simulink model "slipm3D_zir"  (R2025b)
settings: Solver=ode4  StartTime=0.0  StopTime=t_stop  FixedStep=t_step  RelTol=1e-3
values from neighbouring files (symbols this model uses):
  dx0 = -0.467    [ref_data_zir.m]
  dy0 = 0.467    [ref_data_zir.m]
  t_step = 0.001    [ref_data_zir.m]
  x0 = 0.151    [ref_data_zir.m]
  y0 = 0.05    [ref_data_zir.m]
settings Model: Creator=Admin  LastModifiedBy=Vishal
settings OptimizationCC: ReuseModelBlockBuffer=off
settings RTWCC: GPUComputeCapability=3.5

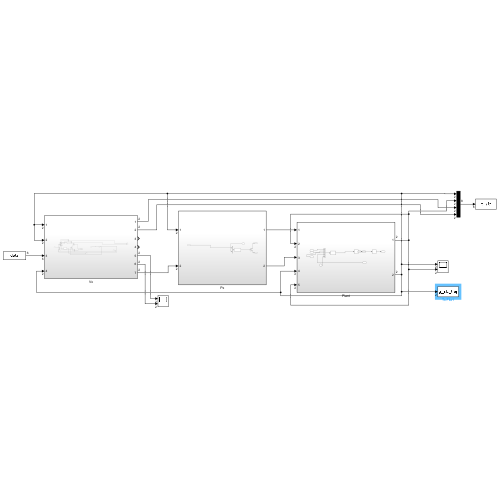
[thumbnail: Simulink's stored preview of the top-level diagram]
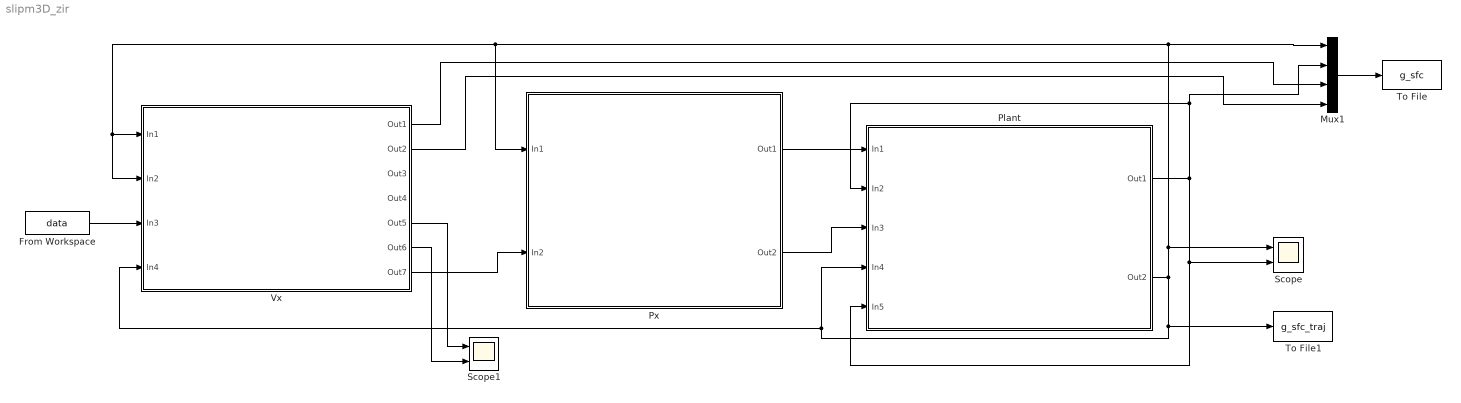
== system slipm3D_zir ==
  From Workspace : FromWorkspace  VariableName=data  OutDataTypeStr=double  SampleTime=t_step
  Mux1 : Mux
  Plant : Subsystem
  Px : Subsystem
  Scope : Scope  NumInputPorts=2
      settings: ActiveDisplayYMinimum=-0.064169644280956978  ActiveDisplayYMaximum=1.077526798528613
  Scope1 : Scope  NumInputPorts=2
      settings: ActiveDisplayYMinimum=0.08202  ActiveDisplayYMaximum=0.48484
  To File : ToFile  Filename=g_sfc  MatrixName=states_sfc
  To File1 : ToFile  Filename=g_sfc_traj  MatrixName=staj
  Vx : Subsystem
  wires:
  Mux1/1 -> To File/1
  Plant/2(Out2) -> To File1/1, Plant/4(In4), Vx/4(In4), Scope/1, Mux1/1, Vx/1(In1), Vx/2(In2), Px/1(In1)
  Plant/1(Out1) -> Plant/5(In5), Scope/2, Plant/2(In2), Mux1/2
  Px/1(Out1) -> Plant/1(In1)
  Px/2(Out2) -> Plant/3(In3)
  From Workspace/1 -> Vx/3(In3)
  Vx/1(Out1) -> Mux1/3
  Vx/2(Out2) -> Mux1/4
  Vx/5(Out5) -> Scope1/1
  Vx/6(Out6) -> Scope1/2
  Vx/7(Out7) -> Px/2(In2)

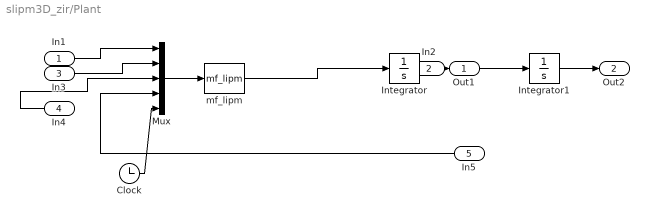
== system slipm3D_zir/Plant ==
  In1 : Inport
  In2 : Inport  Port=2
  In3 : Inport  Port=3
  In4 : Inport  Port=4
  In5 : Inport  Port=5
  Clock : Clock
  Integrator : Integrator  InitialCondition=[dx0,dy0]
  Integrator1 : Integrator  InitialCondition=[x0,y0]
  Mux : Mux  Inputs=5
  mf_lipm : MATLABFcn  MATLABFcn=mf_lipm  OutputDimensions=2
  Out1 : Outport
  Out2 : Outport  Port=2
  wires:
  Clock/1 -> Mux/5
  In4/1 -> Mux/3
  mf_lipm/1 -> Integrator/1
  Integrator/1 -> Out1/1
  In1/1 -> Mux/1
  Integrator1/1 -> Out2/1
  Mux/1 -> mf_lipm/1
  In3/1 -> Mux/2
  In5/1 -> Mux/4
  In2/1 -> Integrator1/1

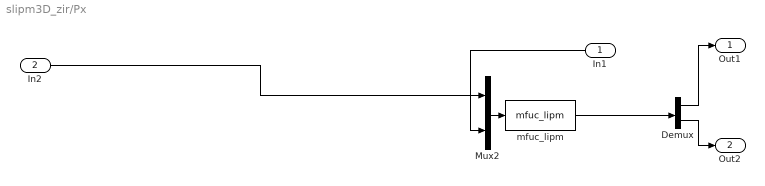
== system slipm3D_zir/Px ==
  In1 : Inport
  In2 : Inport  Port=2
  Demux : Demux  Outputs=2
  Mux2 : Mux  Inputs=2
  mfuc_lipm : MATLABFcn  MATLABFcn=mfuc_lipm  OutputDimensions=2
  Out1 : Outport
  Out2 : Outport  Port=2
  wires:
  In2/1 -> Mux2/1
  In1/1 -> Mux2/2
  Mux2/1 -> mfuc_lipm/1
  mfuc_lipm/1 -> Demux/1
  Demux/2 -> Out2/1
  Demux/1 -> Out1/1

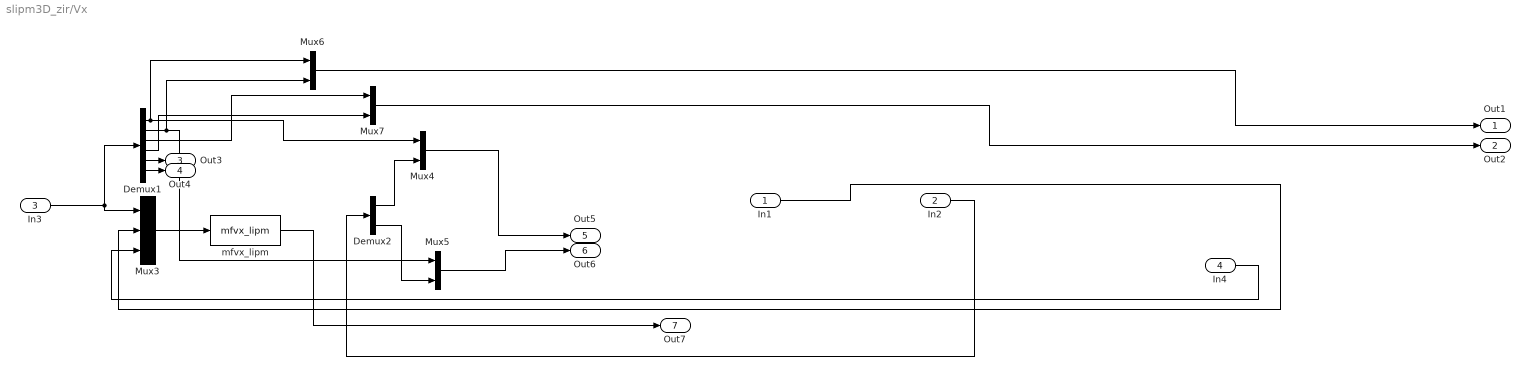
== system slipm3D_zir/Vx ==
  In1 : Inport
  In2 : Inport  Port=2
  In3 : Inport  Port=3
  In4 : Inport  Port=4
  Demux1 : Demux  Outputs=6
  Demux2 : Demux  Outputs=2
  Mux3 : Mux  Inputs=3
  Mux{4..7} (4 alike) : Mux  Inputs=2
  mfvx_lipm : MATLABFcn  MATLABFcn=mfvx_lipm  OutputDimensions=2
  Out1 : Outport
  Out2 : Outport  Port=2
  Out3 : Outport  Port=3
  Out4 : Outport  Port=4
  Out5 : Outport  Port=5
  Out6 : Outport  Port=6
  Out7 : Outport  Port=7
  wires:
  In4/1 -> Mux3/3
  Demux1/6 -> Out4/1
  Demux1/3 -> Mux7/1
  Demux1/1 -> Mux6/1, Mux4/1
  Mux3/1 -> mfvx_lipm/1
  Demux2/2 -> Mux5/2
  In1/1 -> Mux3/2
  In3/1 -> Demux1/1, Mux3/1
  Demux1/4 -> Mux7/2
  Demux2/1 -> Mux4/2
  Demux1/2 -> Mux6/2, Mux5/1
  Mux5/1 -> Out6/1
  Mux7/1 -> Out2/1
  In2/1 -> Demux2/1
  Mux4/1 -> Out5/1
  Mux6/1 -> Out1/1
  mfvx_lipm/1 -> Out7/1
  Demux1/5 -> Out3/1
